simulink model "P702_NI_SoftECU"  (R2019a)
settings: Solver=ode1  StartTime=0.0  StopTime=Inf  FixedStep=0.001  RelTol=1e-3  EnableMultiTasking=on
PreLoadFcn:
  | run '.\VeriStand_BlockSet\NIVeriStandAddPaths.m'
undefined symbols (not defined in the file or in its folder): magnitude
libraries: simulink x83, simulink_extras x1
(part 40 of 76)

== system P702_NI_SoftECU/Output/SoftECULogic_NIXNET_CAN_FD1/WheelSpeed ==
  in : Inport
  WhlFl_W_Meas : S-Function  Priority=4  FunctionName=NIVeriStandIO  Parameters=width dtype portnum stime stype btype  SFunctionDeploymentMode=off  EnableBusSupport=off  mask(NI VeriStand Outport){portnum=4, width=-1, stime=-1, dtype=auto, stype=auto, btype=0}
      mask prompts: portnum "Port number:"; width "Port dimensions (-1 for dynamically sized):"; stime "Sample time (-1 for inherited):"; dtype "Data type:"; stype "Signal type:"; btype "Block type:"
      mask help: Use this outport on any level of nested subsystems to allow NI VeriStand software to map signals to it.
      mask init:
      | NIVeriStandIO_init;
      settings: CopyFcn=NIVeriStand_MDL_functions('', 'IO_copy');  DeleteFcn=NIVeriStand_MDL_functions('', 'IO_delete');  MoveFcn=set_param(gcb, 'Mask', 'on');
      mask Callback portnum: NIVeriStand_MDL_functions('', 'IO_setportnum');
      mask TypeOptions dtype: auto | double | single | int8 | uint8 | int16 | uint16 | int32 | uint32 | boolean
      mask Callback dtype: NIVeriStand_MDL_functions('', 'IO_booleansignal');
      mask TypeOptions stype: auto | real | complex
      mask Display:
      | patch([-x x], [-y y], [.90980 .81960 .32156]);
      | plot([xrad -x x xrad], [yrad -y y yrad]);
      | fprintf('NI Out%d', portnum);
  WhlFr_W_Meas : S-Function  Priority=3  FunctionName=NIVeriStandIO  Parameters=width dtype portnum stime stype btype  SFunctionDeploymentMode=off  EnableBusSupport=off  mask(NI VeriStand Outport){portnum=3, width=-1, stime=-1, dtype=auto, stype=auto, btype=0}
      mask prompts: portnum "Port number:"; width "Port dimensions (-1 for dynamically sized):"; stime "Sample time (-1 for inherited):"; dtype "Data type:"; stype "Signal type:"; btype "Block type:"
      mask help: Use this outport on any level of nested subsystems to allow NI VeriStand software to map signals to it.
      mask init:
      | NIVeriStandIO_init;
      settings: CopyFcn=NIVeriStand_MDL_functions('', 'IO_copy');  DeleteFcn=NIVeriStand_MDL_functions('', 'IO_delete');  MoveFcn=set_param(gcb, 'Mask', 'on');
      mask Callback portnum: NIVeriStand_MDL_functions('', 'IO_setportnum');
      mask TypeOptions dtype: auto | double | single | int8 | uint8 | int16 | uint16 | int32 | uint32 | boolean
      mask Callback dtype: NIVeriStand_MDL_functions('', 'IO_booleansignal');
      mask TypeOptions stype: auto | real | complex
      mask Display:
      | patch([-x x], [-y y], [.90980 .81960 .32156]);
      | plot([xrad -x x xrad], [yrad -y y yrad]);
      | fprintf('NI Out%d', portnum);
  WhlRl_W_Meas : S-Function  Priority=2  FunctionName=NIVeriStandIO  Parameters=width dtype portnum stime stype btype  SFunctionDeploymentMode=off  EnableBusSupport=off  mask(NI VeriStand Outport){portnum=2, width=-1, stime=-1, dtype=auto, stype=auto, btype=0}
      mask prompts: portnum "Port number:"; width "Port dimensions (-1 for dynamically sized):"; stime "Sample time (-1 for inherited):"; dtype "Data type:"; stype "Signal type:"; btype "Block type:"
      mask help: Use this outport on any level of nested subsystems to allow NI VeriStand software to map signals to it.
      mask init:
      | NIVeriStandIO_init;
      settings: CopyFcn=NIVeriStand_MDL_functions('', 'IO_copy');  DeleteFcn=NIVeriStand_MDL_functions('', 'IO_delete');  MoveFcn=set_param(gcb, 'Mask', 'on');
      mask Callback portnum: NIVeriStand_MDL_functions('', 'IO_setportnum');
      mask TypeOptions dtype: auto | double | single | int8 | uint8 | int16 | uint16 | int32 | uint32 | boolean
      mask Callback dtype: NIVeriStand_MDL_functions('', 'IO_booleansignal');
      mask TypeOptions stype: auto | real | complex
      mask Display:
      | patch([-x x], [-y y], [.90980 .81960 .32156]);
      | plot([xrad -x x xrad], [yrad -y y yrad]);
      | fprintf('NI Out%d', portnum);
  WhlRotatFl_No_Cnt : S-Function  Priority=5  FunctionName=NIVeriStandIO  Parameters=width dtype portnum stime stype btype  SFunctionDeploymentMode=off  EnableBusSupport=off  mask(NI VeriStand Outport){portnum=5, width=-1, stime=-1, dtype=auto, stype=auto, btype=0}
      mask prompts: portnum "Port number:"; width "Port dimensions (-1 for dynamically sized):"; stime "Sample time (-1 for inherited):"; dtype "Data type:"; stype "Signal type:"; btype "Block type:"
      mask help: Use this outport on any level of nested subsystems to allow NI VeriStand software to map signals to it.
      mask init:
      | NIVeriStandIO_init;
      settings: CopyFcn=NIVeriStand_MDL_functions('', 'IO_copy');  DeleteFcn=NIVeriStand_MDL_functions('', 'IO_delete');  MoveFcn=set_param(gcb, 'Mask', 'on');
      mask Callback portnum: NIVeriStand_MDL_functions('', 'IO_setportnum');
      mask TypeOptions dtype: auto | double | single | int8 | uint8 | int16 | uint16 | int32 | uint32 | boolean
      mask Callback dtype: NIVeriStand_MDL_functions('', 'IO_booleansignal');
      mask TypeOptions stype: auto | real | complex
      mask Display:
      | patch([-x x], [-y y], [.90980 .81960 .32156]);
      | plot([xrad -x x xrad], [yrad -y y yrad]);
      | fprintf('NI Out%d', portnum);
  WhlRotatFr_No_Cnt : S-Function  Priority=6  FunctionName=NIVeriStandIO  Parameters=width dtype portnum stime stype btype  SFunctionDeploymentMode=off  EnableBusSupport=off  mask(NI VeriStand Outport){portnum=6, width=-1, stime=-1, dtype=auto, stype=auto, btype=0}
      mask prompts: portnum "Port number:"; width "Port dimensions (-1 for dynamically sized):"; stime "Sample time (-1 for inherited):"; dtype "Data type:"; stype "Signal type:"; btype "Block type:"
      mask help: Use this outport on any level of nested subsystems to allow NI VeriStand software to map signals to it.
      mask init:
      | NIVeriStandIO_init;
      settings: CopyFcn=NIVeriStand_MDL_functions('', 'IO_copy');  DeleteFcn=NIVeriStand_MDL_functions('', 'IO_delete');  MoveFcn=set_param(gcb, 'Mask', 'on');
      mask Callback portnum: NIVeriStand_MDL_functions('', 'IO_setportnum');
      mask TypeOptions dtype: auto | double | single | int8 | uint8 | int16 | uint16 | int32 | uint32 | boolean
      mask Callback dtype: NIVeriStand_MDL_functions('', 'IO_booleansignal');
      mask TypeOptions stype: auto | real | complex
      mask Display:
      | patch([-x x], [-y y], [.90980 .81960 .32156]);
      | plot([xrad -x x xrad], [yrad -y y yrad]);
      | fprintf('NI Out%d', portnum);
  WhlRotatRl_No_Cnt : S-Function  Priority=7  FunctionName=NIVeriStandIO  Parameters=width dtype portnum stime stype btype  SFunctionDeploymentMode=off  EnableBusSupport=off  mask(NI VeriStand Outport){portnum=7, width=-1, stime=-1, dtype=auto, stype=auto, btype=0}
      mask prompts: portnum "Port number:"; width "Port dimensions (-1 for dynamically sized):"; stime "Sample time (-1 for inherited):"; dtype "Data type:"; stype "Signal type:"; btype "Block type:"
      mask help: Use this outport on any level of nested subsystems to allow NI VeriStand software to map signals to it.
      mask init:
      | NIVeriStandIO_init;
      settings: CopyFcn=NIVeriStand_MDL_functions('', 'IO_copy');  DeleteFcn=NIVeriStand_MDL_functions('', 'IO_delete');  MoveFcn=set_param(gcb, 'Mask', 'on');
      mask Callback portnum: NIVeriStand_MDL_functions('', 'IO_setportnum');
      mask TypeOptions dtype: auto | double | single | int8 | uint8 | int16 | uint16 | int32 | uint32 | boolean
      mask Callback dtype: NIVeriStand_MDL_functions('', 'IO_booleansignal');
      mask TypeOptions stype: auto | real | complex
      mask Display:
      | patch([-x x], [-y y], [.90980 .81960 .32156]);
      | plot([xrad -x x xrad], [yrad -y y yrad]);
      | fprintf('NI Out%d', portnum);
  WhlRotatRr_No_Cnt : S-Function  Priority=8  FunctionName=NIVeriStandIO  Parameters=width dtype portnum stime stype btype  SFunctionDeploymentMode=off  EnableBusSupport=off  mask(NI VeriStand Outport){portnum=8, width=-1, stime=-1, dtype=auto, stype=auto, btype=0}
      mask prompts: portnum "Port number:"; width "Port dimensions (-1 for dynamically sized):"; stime "Sample time (-1 for inherited):"; dtype "Data type:"; stype "Signal type:"; btype "Block type:"
      mask help: Use this outport on any level of nested subsystems to allow NI VeriStand software to map signals to it.
      mask init:
      | NIVeriStandIO_init;
      settings: CopyFcn=NIVeriStand_MDL_functions('', 'IO_copy');  DeleteFcn=NIVeriStand_MDL_functions('', 'IO_delete');  MoveFcn=set_param(gcb, 'Mask', 'on');
      mask Callback portnum: NIVeriStand_MDL_functions('', 'IO_setportnum');
      mask TypeOptions dtype: auto | double | single | int8 | uint8 | int16 | uint16 | int32 | uint32 | boolean
      mask Callback dtype: NIVeriStand_MDL_functions('', 'IO_booleansignal');
      mask TypeOptions stype: auto | real | complex
      mask Display:
      | patch([-x x], [-y y], [.90980 .81960 .32156]);
      | plot([xrad -x x xrad], [yrad -y y yrad]);
      | fprintf('NI Out%d', portnum);
  WhlRr_W_Meas : S-Function  Priority=1  FunctionName=NIVeriStandIO  Parameters=width dtype portnum stime stype btype  SFunctionDeploymentMode=off  EnableBusSupport=off  mask(NI VeriStand Outport){portnum=1, width=-1, stime=-1, dtype=auto, stype=auto, btype=0}
      mask prompts: portnum "Port number:"; width "Port dimensions (-1 for dynamically sized):"; stime "Sample time (-1 for inherited):"; dtype "Data type:"; stype "Signal type:"; btype "Block type:"
      mask help: Use this outport on any level of nested subsystems to allow NI VeriStand software to map signals to it.
      mask init:
      | NIVeriStandIO_init;
      settings: CopyFcn=NIVeriStand_MDL_functions('', 'IO_copy');  DeleteFcn=NIVeriStand_MDL_functions('', 'IO_delete');  MoveFcn=set_param(gcb, 'Mask', 'on');
      mask Callback portnum: NIVeriStand_MDL_functions('', 'IO_setportnum');
      mask TypeOptions dtype: auto | double | single | int8 | uint8 | int16 | uint16 | int32 | uint32 | boolean
      mask Callback dtype: NIVeriStand_MDL_functions('', 'IO_booleansignal');
      mask TypeOptions stype: auto | real | complex
      mask Display:
      | patch([-x x], [-y y], [.90980 .81960 .32156]);
      | plot([xrad -x x xrad], [yrad -y y yrad]);
      | fprintf('NI Out%d', portnum);
  busselector : BusSelector  OutputSignals=Soft_ABS.WheelSpeed.WhlRr_W_Meas,Soft_ABS.WheelSpeed.WhlRl_W_Meas,Soft_ABS.WheelSpeed.WhlFr_W_Meas,Soft_ABS.WheelSpeed.WhlFl_W_Meas,Soft_ABS.WheelSpeed.WhlRotatFl_No_Cnt,Soft_ABS.WheelSpeed.WhlRotatFr_No_Cnt,Soft_ABS.WheelSpeed.WhlRotatRl_No_Cnt,Soft_ABS.WheelSpeed.WhlRotatRr_No_Cnt
  dt_WhlFl_W_Meas{,1..4} (5 alike) : DataTypeConversion  RndMeth=Zero
  dt_WhlFr_W_Meas : DataTypeConversion  RndMeth=Zero
  dt_WhlRl_W_Meas : DataTypeConversion  RndMeth=Zero
  dt_WhlRr_W_Meas : DataTypeConversion  RndMeth=Zero
  wires:
  in/1 -> busselector/1
  busselector/1 -> dt_WhlRr_W_Meas/1  "<WhlRr_W_Meas>"
  dt_WhlRr_W_Meas/1 -> WhlRr_W_Meas/1  "WhlRr_W_Meas"
  busselector/2 -> dt_WhlRl_W_Meas/1  "<WhlRl_W_Meas>"
  dt_WhlRl_W_Meas/1 -> WhlRl_W_Meas/1  "WhlRl_W_Meas"
  busselector/3 -> dt_WhlFr_W_Meas/1  "<WhlFr_W_Meas>"
  dt_WhlFr_W_Meas/1 -> WhlFr_W_Meas/1  "WhlFr_W_Meas"
  busselector/4 -> dt_WhlFl_W_Meas/1  "<WhlFl_W_Meas>"
  dt_WhlFl_W_Meas/1 -> WhlFl_W_Meas/1  "WhlFl_W_Meas"
  dt_WhlFl_W_Meas1/1 -> WhlRotatFr_No_Cnt/1  "<WhlRotatFr_No_Cnt>"
  dt_WhlFl_W_Meas2/1 -> WhlRotatFl_No_Cnt/1  "<WhlRotatFl_No_Cnt>"
  dt_WhlFl_W_Meas3/1 -> WhlRotatRr_No_Cnt/1  "<WhlRotatRr_No_Cnt>"
  dt_WhlFl_W_Meas4/1 -> WhlRotatRl_No_Cnt/1  "<WhlRotatRl_No_Cnt>"
  busselector/7 -> dt_WhlFl_W_Meas3/1  "<WhlRotatRl_No_Cnt>"
  busselector/6 -> dt_WhlFl_W_Meas2/1  "<WhlRotatFr_No_Cnt>"
  busselector/5 -> dt_WhlFl_W_Meas1/1  "<WhlRotatFl_No_Cnt>"
  busselector/8 -> dt_WhlFl_W_Meas4/1  "<WhlRotatRr_No_Cnt>"

== system P702_NI_SoftECU/Output/SoftECULogic_NIXNET_CAN_FD1/Yaw_Data ==
  in : Inport
  VehRolWActl_D_Qf : S-Function  Priority=2  FunctionName=NIVeriStandIO  Parameters=width dtype portnum stime stype btype  SFunctionDeploymentMode=off  EnableBusSupport=off  mask(NI VeriStand Outport){portnum=2, width=-1, stime=-1, dtype=auto, stype=auto, btype=0}
      mask prompts: portnum "Port number:"; width "Port dimensions (-1 for dynamically sized):"; stime "Sample time (-1 for inherited):"; dtype "Data type:"; stype "Signal type:"; btype "Block type:"
      mask help: Use this outport on any level of nested subsystems to allow NI VeriStand software to map signals to it.
      mask init:
      | NIVeriStandIO_init;
      settings: CopyFcn=NIVeriStand_MDL_functions('', 'IO_copy');  DeleteFcn=NIVeriStand_MDL_functions('', 'IO_delete');  MoveFcn=set_param(gcb, 'Mask', 'on');
      mask Callback portnum: NIVeriStand_MDL_functions('', 'IO_setportnum');
      mask TypeOptions dtype: auto | double | single | int8 | uint8 | int16 | uint16 | int32 | uint32 | boolean
      mask Callback dtype: NIVeriStand_MDL_functions('', 'IO_booleansignal');
      mask TypeOptions stype: auto | real | complex
      mask Display:
      | patch([-x x], [-y y], [.90980 .81960 .32156]);
      | plot([xrad -x x xrad], [yrad -y y yrad]);
      | fprintf('NI Out%d', portnum);
  VehRol_W_Actl : S-Function  Priority=3  FunctionName=NIVeriStandIO  Parameters=width dtype portnum stime stype btype  SFunctionDeploymentMode=off  EnableBusSupport=off  mask(NI VeriStand Outport){portnum=3, width=-1, stime=-1, dtype=auto, stype=auto, btype=0}
      mask prompts: portnum "Port number:"; width "Port dimensions (-1 for dynamically sized):"; stime "Sample time (-1 for inherited):"; dtype "Data type:"; stype "Signal type:"; btype "Block type:"
      mask help: Use this outport on any level of nested subsystems to allow NI VeriStand software to map signals to it.
      mask init:
      | NIVeriStandIO_init;
      settings: CopyFcn=NIVeriStand_MDL_functions('', 'IO_copy');  DeleteFcn=NIVeriStand_MDL_functions('', 'IO_delete');  MoveFcn=set_param(gcb, 'Mask', 'on');
      mask Callback portnum: NIVeriStand_MDL_functions('', 'IO_setportnum');
      mask TypeOptions dtype: auto | double | single | int8 | uint8 | int16 | uint16 | int32 | uint32 | boolean
      mask Callback dtype: NIVeriStand_MDL_functions('', 'IO_booleansignal');
      mask TypeOptions stype: auto | real | complex
      mask Display:
      | patch([-x x], [-y y], [.90980 .81960 .32156]);
      | plot([xrad -x x xrad], [yrad -y y yrad]);
      | fprintf('NI Out%d', portnum);
  VehRollYawW_No_Cs : S-Function  Priority=4  FunctionName=NIVeriStandIO  Parameters=width dtype portnum stime stype btype  SFunctionDeploymentMode=off  EnableBusSupport=off  mask(NI VeriStand Outport){portnum=4, width=-1, stime=-1, dtype=auto, stype=auto, btype=0}
      mask prompts: portnum "Port number:"; width "Port dimensions (-1 for dynamically sized):"; stime "Sample time (-1 for inherited):"; dtype "Data type:"; stype "Signal type:"; btype "Block type:"
      mask help: Use this outport on any level of nested subsystems to allow NI VeriStand software to map signals to it.
      mask init:
      | NIVeriStandIO_init;
      settings: CopyFcn=NIVeriStand_MDL_functions('', 'IO_copy');  DeleteFcn=NIVeriStand_MDL_functions('', 'IO_delete');  MoveFcn=set_param(gcb, 'Mask', 'on');
      mask Callback portnum: NIVeriStand_MDL_functions('', 'IO_setportnum');
      mask TypeOptions dtype: auto | double | single | int8 | uint8 | int16 | uint16 | int32 | uint32 | boolean
      mask Callback dtype: NIVeriStand_MDL_functions('', 'IO_booleansignal');
      mask TypeOptions stype: auto | real | complex
      mask Display:
      | patch([-x x], [-y y], [.90980 .81960 .32156]);
      | plot([xrad -x x xrad], [yrad -y y yrad]);
      | fprintf('NI Out%d', portnum);
  VehRollYaw_No_Cnt : S-Function  Priority=5  FunctionName=NIVeriStandIO  Parameters=width dtype portnum stime stype btype  SFunctionDeploymentMode=off  EnableBusSupport=off  mask(NI VeriStand Outport){portnum=5, width=-1, stime=-1, dtype=auto, stype=auto, btype=0}
      mask prompts: portnum "Port number:"; width "Port dimensions (-1 for dynamically sized):"; stime "Sample time (-1 for inherited):"; dtype "Data type:"; stype "Signal type:"; btype "Block type:"
      mask help: Use this outport on any level of nested subsystems to allow NI VeriStand software to map signals to it.
      mask init:
      | NIVeriStandIO_init;
      settings: CopyFcn=NIVeriStand_MDL_functions('', 'IO_copy');  DeleteFcn=NIVeriStand_MDL_functions('', 'IO_delete');  MoveFcn=set_param(gcb, 'Mask', 'on');
      mask Callback portnum: NIVeriStand_MDL_functions('', 'IO_setportnum');
      mask TypeOptions dtype: auto | double | single | int8 | uint8 | int16 | uint16 | int32 | uint32 | boolean
      mask Callback dtype: NIVeriStand_MDL_functions('', 'IO_booleansignal');
      mask TypeOptions stype: auto | real | complex
      mask Display:
      | patch([-x x], [-y y], [.90980 .81960 .32156]);
      | plot([xrad -x x xrad], [yrad -y y yrad]);
      | fprintf('NI Out%d', portnum);
  VehYawWActl_D_Qf : S-Function  Priority=6  FunctionName=NIVeriStandIO  Parameters=width dtype portnum stime stype btype  SFunctionDeploymentMode=off  EnableBusSupport=off  mask(NI VeriStand Outport){portnum=6, width=-1, stime=-1, dtype=auto, stype=auto, btype=0}
      mask prompts: portnum "Port number:"; width "Port dimensions (-1 for dynamically sized):"; stime "Sample time (-1 for inherited):"; dtype "Data type:"; stype "Signal type:"; btype "Block type:"
      mask help: Use this outport on any level of nested subsystems to allow NI VeriStand software to map signals to it.
      mask init:
      | NIVeriStandIO_init;
      settings: CopyFcn=NIVeriStand_MDL_functions('', 'IO_copy');  DeleteFcn=NIVeriStand_MDL_functions('', 'IO_delete');  MoveFcn=set_param(gcb, 'Mask', 'on');
      mask Callback portnum: NIVeriStand_MDL_functions('', 'IO_setportnum');
      mask TypeOptions dtype: auto | double | single | int8 | uint8 | int16 | uint16 | int32 | uint32 | boolean
      mask Callback dtype: NIVeriStand_MDL_functions('', 'IO_booleansignal');
      mask TypeOptions stype: auto | real | complex
      mask Display:
      | patch([-x x], [-y y], [.90980 .81960 .32156]);
      | plot([xrad -x x xrad], [yrad -y y yrad]);
      | fprintf('NI Out%d', portnum);
  VehYaw_W_Actl : S-Function  Priority=1  FunctionName=NIVeriStandIO  Parameters=width dtype portnum stime stype btype  SFunctionDeploymentMode=off  EnableBusSupport=off  mask(NI VeriStand Outport){portnum=1, width=-1, stime=-1, dtype=auto, stype=auto, btype=0}
      mask prompts: portnum "Port number:"; width "Port dimensions (-1 for dynamically sized):"; stime "Sample time (-1 for inherited):"; dtype "Data type:"; stype "Signal type:"; btype "Block type:"
      mask help: Use this outport on any level of nested subsystems to allow NI VeriStand software to map signals to it.
      mask init:
      | NIVeriStandIO_init;
      settings: CopyFcn=NIVeriStand_MDL_functions('', 'IO_copy');  DeleteFcn=NIVeriStand_MDL_functions('', 'IO_delete');  MoveFcn=set_param(gcb, 'Mask', 'on');
      mask Callback portnum: NIVeriStand_MDL_functions('', 'IO_setportnum');
      mask TypeOptions dtype: auto | double | single | int8 | uint8 | int16 | uint16 | int32 | uint32 | boolean
      mask Callback dtype: NIVeriStand_MDL_functions('', 'IO_booleansignal');
      mask TypeOptions stype: auto | real | complex
      mask Display:
      | patch([-x x], [-y y], [.90980 .81960 .32156]);
      | plot([xrad -x x xrad], [yrad -y y yrad]);
      | fprintf('NI Out%d', portnum);
  busselector : BusSelector  OutputSignals=Soft_RCM.Yaw_Data.VehYawWActl_D_Qf,Soft_RCM.Yaw_Data.VehRolWActl_D_Qf,Soft_RCM.Yaw_Data.VehRollYaw_No_Cnt,Soft_RCM.Yaw_Data.VehRollYawW_No_Cs,Soft_RCM.Yaw_Data.VehYaw_W_Actl,Soft_RCM.Yaw_Data.VehRol_W_Actl
  dt_VehRolWActl_D_Qf : DataTypeConversion  RndMeth=Zero
  dt_VehRol_W_Actl : DataTypeConversion  RndMeth=Zero
  dt_VehRollYawW_No_Cs : DataTypeConversion  RndMeth=Zero
  dt_VehRollYaw_No_Cnt : DataTypeConversion  RndMeth=Zero
  dt_VehYawWActl_D_Qf : DataTypeConversion  RndMeth=Zero
  dt_VehYaw_W_Actl : DataTypeConversion  RndMeth=Zero
  wires:
  in/1 -> busselector/1
  busselector/1 -> dt_VehYawWActl_D_Qf/1  "<VehYawWActl_D_Qf>"
  dt_VehYawWActl_D_Qf/1 -> VehYawWActl_D_Qf/1  "VehYawWActl_D_Qf"
  busselector/2 -> dt_VehRolWActl_D_Qf/1  "<VehRolWActl_D_Qf>"
  dt_VehRolWActl_D_Qf/1 -> VehRolWActl_D_Qf/1  "VehRolWActl_D_Qf"
  busselector/3 -> dt_VehRollYaw_No_Cnt/1  "<VehRollYaw_No_Cnt>"
  dt_VehRollYaw_No_Cnt/1 -> VehRollYaw_No_Cnt/1  "VehRollYaw_No_Cnt"
  busselector/4 -> dt_VehRollYawW_No_Cs/1  "<VehRollYawW_No_Cs>"
  dt_VehRollYawW_No_Cs/1 -> VehRollYawW_No_Cs/1  "VehRollYawW_No_Cs"
  busselector/5 -> dt_VehYaw_W_Actl/1  "<VehYaw_W_Actl>"
  dt_VehYaw_W_Actl/1 -> VehYaw_W_Actl/1  "VehYaw_W_Actl"
  busselector/6 -> dt_VehRol_W_Actl/1  "<VehRol_W_Actl>"
  dt_VehRol_W_Actl/1 -> VehRol_W_Actl/1  "VehRol_W_Actl"

== system P702_NI_SoftECU/Output/Subsystem/a//b ==
  Constant : Constant
  x/y : Constant
  Out1 : Outport
  wires:
  Constant/1 -> Out1/1

== system P702_NI_SoftECU/Output/Subsystem/c ==
  In1 : Inport
  Out1 : Outport
  wires:
  In1/1 -> Out1/1

== system P702_NI_SoftECU/Output/Subsystem/d ==
  In1 : Inport
  Out1 : Outport
  wires:
  In1/1 -> Out1/1

== system P702_NI_SoftECU/Output/Subsystem1/CAN_Signal ==
  in_port : Inport
  ABS_ESC : Subsystem
  ADAS : Subsystem
  BCM : Subsystem
  DSMC : Subsystem
  ECM_DIESEL PCM PCM_HEV : Subsystem
  GWM : Subsystem
  PSCM : Subsystem
  RealPCM : Subsystem
  bus_selector : BusSelector  OutputSignals=ADAS,RealPCM,ABS_ESC,PSCM,ECM_DIESEL PCM PCM_HEV,BCM,GWM,DSMC
  wires:
  in_port/1 -> bus_selector/1  "Subsystem1"
  bus_selector/1 -> ADAS/1(in_port)  "<ADAS>"
  bus_selector/2 -> RealPCM/1(in_port)  "<RealPCM>"
  bus_selector/3 -> ABS_ESC/1(in_port)  "<ABS_ESC>"
  bus_selector/4 -> PSCM/1(in_port)  "<PSCM>"
  bus_selector/5 -> ECM_DIESEL PCM PCM_HEV/1(in_port)  "<ECM_DIESEL PCM PCM_HEV>"
  bus_selector/6 -> BCM/1(in_port)  "<BCM>"
  bus_selector/7 -> GWM/1(in_port)  "<GWM>"
  bus_selector/8 -> DSMC/1(in_port)  "<DSMC>"

== system P702_NI_SoftECU/Output/Subsystem1/To_NI_HIL ==
  in_port : Inport
  DSMC : Subsystem
  MRR : Subsystem
  SRR_L : Subsystem
  SRR_R : Subsystem
  Soft_ABS : Subsystem
  Soft_APIM : Terminator
  Soft_BCM : Subsystem
  Soft_CCM : Terminator
  Soft_ECM : Subsystem
  Soft_IPC : Terminator
  Soft_IPMA : Terminator
  Soft_MRR : Subsystem
  Soft_PCM : Subsystem
  Soft_PSCM : Subsystem
  Soft_RCM : Subsystem
  Soft_SCCM : Subsystem
  Soft_TCM : Subsystem
  bus_selector : BusSelector  OutputSignals=Soft_ABS,Soft_PCM,Soft_ECM,Soft_TCM,Soft_PSCM,Soft_RCM,Soft_SCCM,Soft_MRR,Soft_BCM,Soft_IPC,Soft_APIM,Soft_IPMA,Soft_CCM,MRR,SRR_R,SRR_L,DSMC
  wires:
  in_port/1 -> bus_selector/1  "Subsystem1"
  bus_selector/10 -> Soft_IPC/1  "<Soft_IPC>"
  bus_selector/11 -> Soft_APIM/1  "<Soft_APIM>"
  bus_selector/12 -> Soft_IPMA/1  "<Soft_IPMA>"
  bus_selector/13 -> Soft_CCM/1  "<Soft_CCM>"
  bus_selector/1 -> Soft_ABS/1(in_port)  "<Soft_ABS>"
  bus_selector/2 -> Soft_PCM/1(in_port)  "<Soft_PCM>"
  bus_selector/3 -> Soft_ECM/1(in_port)  "<Soft_ECM>"
  bus_selector/4 -> Soft_TCM/1(in_port)  "<Soft_TCM>"
  bus_selector/5 -> Soft_PSCM/1(in_port)  "<Soft_PSCM>"
  bus_selector/6 -> Soft_RCM/1(in_port)  "<Soft_RCM>"
  bus_selector/7 -> Soft_SCCM/1(in_port)  "<Soft_SCCM>"
  bus_selector/8 -> Soft_MRR/1(in_port)  "<Soft_MRR>"
  bus_selector/9 -> Soft_BCM/1(in_port)  "<Soft_BCM>"
  bus_selector/14 -> MRR/1(in_port)  "<MRR>"
  bus_selector/15 -> SRR_R/1(in_port)  "<SRR_R>"
  bus_selector/16 -> SRR_L/1(in_port)  "<SRR_L>"
  bus_selector/17 -> DSMC/1(in_port)  "<DSMC>"

== system P702_NI_SoftECU/Output/Subsystem2/CAN_Signal ==
  ABS_ESC : Subsystem
  ADAS : Subsystem
  BCM : Subsystem
  DSMC : Subsystem
  ECM_DIESEL PCM PCM_HEV : Subsystem
  GWM : Subsystem
  PSCM : Subsystem
  RealPCM : Subsystem
  bus_creator : BusCreator  Inputs=8
  out_port : Outport
  wires:
  bus_creator/1 -> out_port/1  "Subsystem2"
  ADAS/1(out_port) -> bus_creator/1  "ADAS"
  RealPCM/1(out_port) -> bus_creator/2  "RealPCM"
  ABS_ESC/1(out_port) -> bus_creator/3  "ABS_ESC"
  PSCM/1(out_port) -> bus_creator/4  "PSCM"
  ECM_DIESEL PCM PCM_HEV/1(out_port) -> bus_creator/5  "ECM_DIESEL PCM PCM_HEV"
  BCM/1(out_port) -> bus_creator/6  "BCM"
  GWM/1(out_port) -> bus_creator/7  "GWM"
  DSMC/1(out_port) -> bus_creator/8  "DSMC"

== system P702_NI_SoftECU/Output/Subsystem2/To_NI_HIL ==
  DSMC : Subsystem
  MRR : Subsystem
  SRR_L : Subsystem
  SRR_R : Subsystem
  Soft_ABS : Subsystem
  Soft_APIM : Constant  Value=0
  Soft_BCM : Subsystem
  Soft_CCM : Constant  Value=0
  Soft_ECM : Subsystem
  Soft_IPC : Constant  Value=0
  Soft_IPMA : Constant  Value=0
  Soft_MRR : Subsystem
  Soft_PCM : Subsystem
  Soft_PSCM : Subsystem
  Soft_RCM : Subsystem
  Soft_SCCM : Subsystem
  Soft_TCM : Subsystem
  bus_creator : BusCreator  Inputs=17
  out_port : Outport
  wires:
  bus_creator/1 -> out_port/1  "Subsystem2"
  Soft_IPC/1 -> bus_creator/10  "Soft_IPC"
  Soft_APIM/1 -> bus_creator/11  "Soft_APIM"
  Soft_IPMA/1 -> bus_creator/12  "Soft_IPMA"
  Soft_CCM/1 -> bus_creator/13  "Soft_CCM"
  Soft_ABS/1(out_port) -> bus_creator/1  "Soft_ABS"
  Soft_PCM/1(out_port) -> bus_creator/2  "Soft_PCM"
  Soft_ECM/1(out_port) -> bus_creator/3  "Soft_ECM"
  Soft_TCM/1(out_port) -> bus_creator/4  "Soft_TCM"
  Soft_PSCM/1(out_port) -> bus_creator/5  "Soft_PSCM"
  Soft_RCM/1(out_port) -> bus_creator/6  "Soft_RCM"
  Soft_SCCM/1(out_port) -> bus_creator/7  "Soft_SCCM"
  Soft_MRR/1(out_port) -> bus_creator/8  "Soft_MRR"
  Soft_BCM/1(out_port) -> bus_creator/9  "Soft_BCM"
  MRR/1(out_port) -> bus_creator/14  "MRR"
  SRR_R/1(out_port) -> bus_creator/15  "SRR_R"
  SRR_L/1(out_port) -> bus_creator/16  "SRR_L"
  DSMC/1(out_port) -> bus_creator/17  "DSMC"

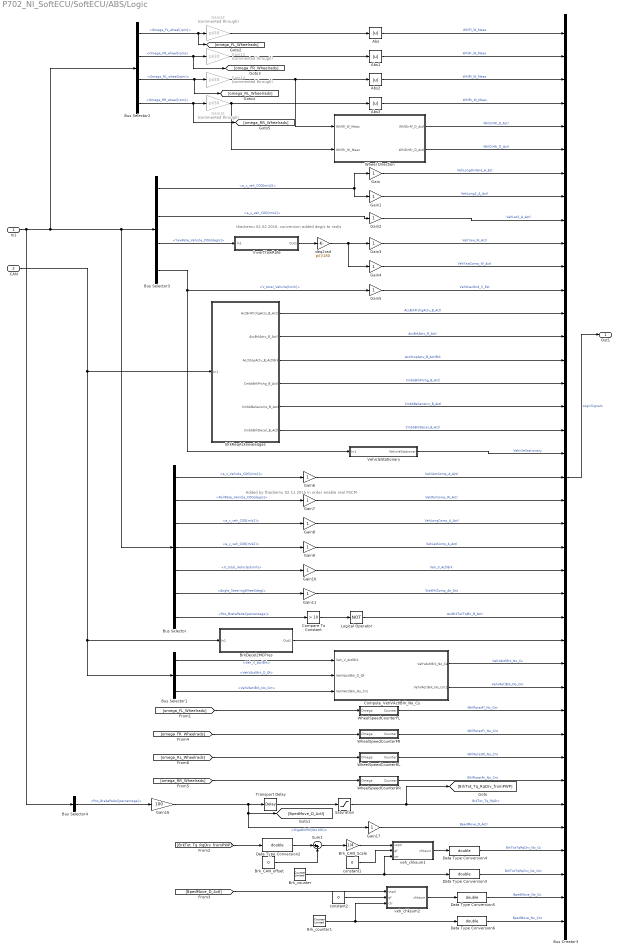
== system P702_NI_SoftECU/SoftECU/ABS/Logic ==
  note: thackemu 02.02.2016: conversion added deg/s to rad/s
  note: Added by thackemu 02.11.2015 in order enable real PSCM
  In1 : Inport
  CAN : Inport  Port=2
  Abs{,1..3} (4 alike) : Abs
  BrkDecel2MCPres : Subsystem
  BrkReqAcknowledges : Subsystem
  Brk_CAN_Scale : Gain  Gain=1/4
  Brk_CAN_offset : Constant  Value=0
  Brk_counter : simulink/Sources/Counter Limited  uplimit=15  tsamp=-1
  Brk_counter1 : simulink/Sources/Counter Limited  uplimit=15  tsamp=-1
  Bus Creator3 : BusCreator  Inputs=39
  Bus Selector : BusSelector  OutputSignals=a_z_Vehicle_COG[m/s2],RollRate_Vehicle_COG[deg/s],a_x_veh_COG[m/s2],a_y_veh_COG[m/s2],V_total_Vehicle[km/h],Angle_SteeringWheel[deg],Pos_BrakePedal[percentage]
  Bus Selector1 : BusSelector  OutputSignals=ABS_ESC.BrakeSysFeatures_0x415.Veh_V_ActlBrk,ABS_ESC.BrakeSysFeatures_0x415.VehVActlBrk_D_Qf,ABS_ESC.BrakeSysFeatures_0x415.VehVActlBrk_No_Cnt
  Bus Selector2 : BusSelector  OutputSignals=Omega_FL_wheel[rpm],Omega_FR_wheel[rpm],Omega_RL_wheel[rpm],Omega_RR_wheel[rpm]
  Bus Selector3 : BusSelector  OutputSignals=a_x_veh_COG[m/s2],a_y_veh_COG[m/s2],YawRate_Vehicle_COG[deg/s],V_total_Vehicle[km/h]
  Bus Selector4 : BusSelector  OutputSignals=Pos_BrakePedal[percentage]
  Compare To Constant : simulink/Logic and Bit Operations/Compare To Constant  relop=>  const=10  OutDataTypeStr=boolean
  Compute_VehVActlBrk_No_Cs : Subsystem
  Data Type Conversion{2..6} (5 alike) : DataTypeConversion  OutDataTypeStr=double
  Gain{,1..11,17} (13 alike) : Gain
  Gain{12..15} (4 alike) : Gain  Commented=through  Gain=pi/30
  Gain16 : Gain  Gain=100
  InvertYawRate : Subsystem
  Logical Operator : Logic  Operator=NOT  AllPortsSameDT=off  OutDataTypeStr=boolean
  Saturation : Saturate  UpperLimit=2000  LowerLimit=0
  Sum1 : Sum  Inputs=|++
  Transport Delay : TransportDelay  DelayTime=0.2  BufferSize=25600  FixedBuffer=on  TransDelayFeedthrough=on
  VehicleStationary : Subsystem
  Wheel Direction : Subsystem
  WheelSpeedCounterFL : Subsystem
  WheelSpeedCounterFR : Subsystem
  WheelSpeedCounterRL : Subsystem
  WheelSpeedCounterRR : Subsystem
  constant1 : Constant  Value=0
  constant2 : Constant  Value=0
  deg2rad : Gain  Gain=pi()/180
  veh_chksum1 : Subsystem
  veh_chksum2 : Subsystem
  Out1 : Outport
  wires:
  Bus Creator3/1 -> Out1/1  "LogicSignals"
  Bus Selector2/1 -> [omega_FL_Wheelrads], Gain12/1  "<Omega_FL_wheel[rpm]>"
  Bus Selector2/2 -> [omega_FR_Wheelrads], Gain13/1  "<Omega_FR_wheel[rpm]>"
  Bus Selector2/3 -> [omega_RL_Wheelrads], Gain14/1  "<Omega_RL_wheel[rpm]>"
  Abs/1 -> Bus Creator3/1  "WhlFl_W_Meas"
  Abs1/1 -> Bus Creator3/2  "WhlFr_W_Meas"
  Abs2/1 -> Bus Creator3/3  "WhlRl_W_Meas"
  Abs3/1 -> Bus Creator3/4  "WhlRr_W_Meas"
  Bus Selector2/4 -> [omega_RR_Wheelrads], Gain15/1  "<Omega_RR_wheel[rpm]>"
  Bus Selector3/2 -> Gain2/1  "<a_y_veh_COG[m/s2]>"
  Bus Selector3/4 -> Gain5/1, VehicleStationary/1(In1)  "<V_total_Vehicle[km/h]>"
  Gain1/1 -> Bus Creator3/8  "VehLong2_A_Actl"
  Gain2/1 -> Bus Creator3/9  "VehLat2_A_Actl"
  Gain3/1 -> Bus Creator3/10  "VehYaw_W_Actl"
  Gain/1 -> Bus Creator3/7  "VehLongOvrGnd_A_Est"
  Gain5/1 -> Bus Creator3/12  "VehOverGnd_V_Est"
  Gain4/1 -> Bus Creator3/11  "VehYawComp_W_Actl"
  Gain6/1 -> Bus Creator3/20  "VehVertComp_A_Actl"
  Gain8/1 -> Bus Creator3/22  "VehLongComp_A_Actl"
  Gain9/1 -> Bus Creator3/23  "VehLatComp_A_Actl"
  Bus Selector/1 -> Gain6/1  "<a_z_Vehicle_COG[m/s2]>"
  Gain7/1 -> Bus Creator3/21  "VehRolComp_W_Actl"
  Bus Selector/2 -> Gain7/1  "<RollRate_Vehicle_COG[deg/s]>"
  Gain10/1 -> Bus Creator3/24  "Veh_V_ActlBrk"
  BrkReqAcknowledges/2(AccBrkActv_B_Actl) -> Bus Creator3/14  "AccBrkActv_B_Actl"
  BrkReqAcknowledges/1(AccBrkPrchgActv_B_Actl) -> Bus Creator3/13  "AccBrkPrchgActv_B_Actl"
  BrkReqAcknowledges/3(AccStopActv_B_ActlBrk) -> Bus Creator3/15  "AccStopActv_B_ActlBrk"
  BrkReqAcknowledges/4(CmbbBrkPrchg_B_Actl) -> Bus Creator3/16  "CmbbBrkPrchg_B_Actl"
  BrkReqAcknowledges/5(CmbbBaSensInc_B_Actl) -> Bus Creator3/17  "CmbbBaSensInc_B_Actl"
  BrkReqAcknowledges/6(CmbbBrkDecel_B_Actl) -> Bus Creator3/18  "CmbbBrkDecel_B_Actl"
  VehicleStationary/1(VehicleStationary) -> Bus Creator3/19  "VehicleStationary"
  deg2rad/1 -> Gain4/1, Gain3/1
  Bus Selector3/3 -> InvertYawRate/1(In1)  "<YawRate_Vehicle_COG[deg/s]>"
  InvertYawRate/1(Out1) -> deg2rad/1
  Wheel Direction/1(WhlDirRl_D_Actl) -> Bus Creator3/5  "WhlDirRl_D_Actl"
  Wheel Direction/2(WhlDirRr_D_Actl) -> Bus Creator3/6  "WhlDirRr_D_Actl"
  Bus Selector3/1 -> Gain1/1, Gain/1  "<a_x_veh_COG[m/s2]>"
  Gain11/1 -> Bus Creator3/25  "SteWhlComp_An_Est"
  Compare To Constant/1 -> Logical Operator/1
  Logical Operator/1 -> Bus Creator3/26  "AccBrkTotTqMn_B_Actl"
  In1/1 -> Bus Selector4/1, Bus Selector2/1, Bus Selector/1, Bus Selector3/1
  Gain12/1 -> Abs/1
  Gain13/1 -> Abs1/1
  Gain14/1 -> Wheel Direction/1(WhlRl_W_Meas), Abs2/1
  Gain15/1 -> Wheel Direction/2(WhlRr_W_Meas), Abs3/1
  CAN/1 -> BrkReqAcknowledges/1(In1), Bus Selector1/1, BrkDecel2MCPres/1(In1)
  Bus Selector/3 -> Gain8/1  "<a_x_veh_COG[m/s2]>"
  Bus Selector/4 -> Gain9/1  "<a_y_veh_COG[m/s2]>"
  Bus Selector/5 -> Gain10/1  "<V_total_Vehicle[km/h]>"
  Bus Selector/6 -> Gain11/1  "<Angle_SteeringWheel[deg]>"
  Bus Selector/7 -> Compare To Constant/1  "<Pos_BrakePedal[percentage]>"
  BrkDecel2MCPres/1(Out1) -> Bus Creator3/27
  Bus Selector1/1 -> Compute_VehVActlBrk_No_Cs/1(Veh_V_ActlBrk)  "<Veh_V_ActlBrk>"
  Bus Selector1/2 -> Compute_VehVActlBrk_No_Cs/2(VehVActlBrk_D_Qf)  "<VehVActlBrk_D_Qf>"
  Bus Selector1/3 -> Compute_VehVActlBrk_No_Cs/3(VehVActlBrk_No_Cnt)  "<VehVActlBrk_No_Cnt>"
  Compute_VehVActlBrk_No_Cs/1(VehVActlBrk_No_Cs) -> Bus Creator3/28  "VehVActlBrk_No_Cs"
  Compute_VehVActlBrk_No_Cs/2(VehVActlBrk_No_Cnt1) -> Bus Creator3/29  "VehVActlBrk_No_Cnt"
  WheelSpeedCounterFL/1(Counter) -> Bus Creator3/30  "WhlRotatFl_No_Cnt"
  [omega_FL_Wheelrads] -> WheelSpeedCounterFL/1(Omega)
  [omega_RR_Wheelrads] -> WheelSpeedCounterRR/1(Omega)
  WheelSpeedCounterFR/1(Counter) -> Bus Creator3/31  "WhlRotatFr_No_Cnt"
  [omega_RL_Wheelrads] -> WheelSpeedCounterRL/1(Omega)
  WheelSpeedCounterRL/1(Counter) -> Bus Creator3/32  "WhlRotatRl_No_Cnt"
  WheelSpeedCounterRR/1(Counter) -> Bus Creator3/33  "WhlRotatRr_No_Cnt"
  [omega_FR_Wheelrads] -> WheelSpeedCounterFR/1(Omega)
  Bus Selector4/1 -> Gain16/1  "<Pos_BrakePedal[percentage]>"
  Transport Delay/1 -> Saturation/1
  Gain16/1 -> Gain17/1, [BpedMove_D_Actl], Transport Delay/1  "<GigaBrkPdl[0to10K]>"
  Gain17/1 -> Bus Creator3/35  "BpedMove_D_Actl"
  Saturation/1 -> Bus Creator3/34, [BrkTot_Tq_RqDrv_fromPWP]  "BrkTot_Tq_RqDrv"
  veh_chksum1/1(chksum) -> Data Type Conversion4/1
  veh_chksum2/1(chksum) -> Data Type Conversion5/1
  Data Type Conversion5/1 -> Bus Creator3/38  "BpedMove_No_Cs"
  constant1/1 -> veh_chksum1/2(qf)
  [BrkTot_Tq_RqDrv_fromPWP] -> Data Type Conversion2/1
  Data Type Conversion2/1 -> Sum1/1
  Sum1/1 -> Brk_CAN_Scale/1
  Brk_counter1/1 -> veh_chksum2/3(ctr), Data Type Conversion6/1
  Data Type Conversion3/1 -> Bus Creator3/37  "BrkTotTqRqDrv_No_Cnt"
  Data Type Conversion6/1 -> Bus Creator3/39  "BpedMove_No_Cnt"
  constant2/1 -> veh_chksum2/2(qf)
  Brk_CAN_offset/1 -> Sum1/2
  Brk_counter/1 -> veh_chksum1/3(ctr), Data Type Conversion3/1
  Data Type Conversion4/1 -> Bus Creator3/36  "BrkTotTqRqDrv_No_Cs"
  [BpedMove_D_Actl] -> veh_chksum2/1(vspd)
  Brk_CAN_Scale/1 -> veh_chksum1/1(vspd)

== system P702_NI_SoftECU/SoftECU/ABS/Mapping ==
  In1 : Inport
  ABS_BrkBst_Data : Subsystem
  Accel_Data : Subsystem
  BrakeSnData_3 : Subsystem
  BrakeSnData_4 : Subsystem
  BrakeSnData_5 : Subsystem
  BrakeSysFeatures : Subsystem
  BrakeSysFeatures_2 : Subsystem
  Bus Creator1 : BusCreator  Inputs=12
  DesiredTorqBrk : Subsystem
  ToCarSim : Subsystem
  WheelData : Subsystem
  WheelSpeed : Subsystem
  Yaw_Data : Subsystem
  Out1 : Outport
  wires:
  Bus Creator1/1 -> Out1/1
  WheelSpeed/1(Out1) -> Bus Creator1/1  "WheelSpeed"
  WheelData/1(Out1) -> Bus Creator1/2  "WheelData"
  BrakeSysFeatures/1(Out1) -> Bus Creator1/8  "BrakeSysFeatures"
  BrakeSnData_4/1(Out1) -> Bus Creator1/7  "BrakeSnData_4"
  DesiredTorqBrk/1(Out1) -> Bus Creator1/6  "DesiredTorqBrk"
  BrakeSnData_3/1(Out1) -> Bus Creator1/5  "BrakeSnData_3"
  Yaw_Data/1(Out1) -> Bus Creator1/4  "Yaw_Data"
  Accel_Data/1(Out1) -> Bus Creator1/3  "Accel_Data"
  In1/1 -> BrakeSysFeatures_2/1(In1), ABS_BrkBst_Data/1(In1), ToCarSim/1(In1), BrakeSnData_5/1(In1), BrakeSysFeatures/1(In1), BrakeSnData_4/1(In1), DesiredTorqBrk/1(In1), BrakeSnData_3/1(In1), Yaw_Data/1(In1), Accel_Data/1(In1), WheelData/1(In1), WheelSpeed/1(In1)
  BrakeSnData_5/1(Out1) -> Bus Creator1/9  "BrakeSnData_5"
  ToCarSim/1(Out1) -> Bus Creator1/10
  ABS_BrkBst_Data/1(Out1) -> Bus Creator1/11  "ABS_BrkBst_Data"
  BrakeSysFeatures_2/1(Out1) -> Bus Creator1/12  "BrakeSysFeatures_2"

== system P702_NI_SoftECU/SoftECU/BCM/Logic ==
  In1 : Inport
  Bus Creator : BusCreator  Inputs=3
  GGCC_Config_Mgmt_ID : Subsystem
  IgnitionState : Subsystem
  OdometerValues : Subsystem
  Out1 : Outport
  wires:
  Bus Creator/1 -> Out1/1  "LogicSignals"
  OdometerValues/1(Out) -> Bus Creator/1
  GGCC_Config_Mgmt_ID/1(Out1) -> Bus Creator/3
  IgnitionState/1(Out) -> Bus Creator/2
  In1/1 -> OdometerValues/1(In), IgnitionState/1(In)

== system P702_NI_SoftECU/SoftECU/BCM/Mapping ==
  In1 : Inport
  BodyEngGateway_2 : Subsystem
  BodyInfo_3 : Subsystem
  Bus Creator : BusCreator  Inputs=7
  Cluster_Info1 : Subsystem
  GGCC_Config_Mgmt_ID : Subsystem
  Gear_Shift_By_Wire : Subsystem
  KeyStates : Subsystem
  Personality_BCM2_Data : Subsystem
  Out1 : Outport
  wires:
  Cluster_Info1/1(Out) -> Bus Creator/2
  BodyInfo_3/1(Out) -> Bus Creator/3
  GGCC_Config_Mgmt_ID/1(Out1) -> Bus Creator/4
  KeyStates/1(Out) -> Bus Creator/1
  In1/1 -> Gear_Shift_By_Wire/1(In1), BodyEngGateway_2/1(In1), GGCC_Config_Mgmt_ID/1(In1), BodyInfo_3/1(In), Cluster_Info1/1(In), KeyStates/1(In)
  Bus Creator/1 -> Out1/1  "MsgSignals"
  BodyEngGateway_2/1(Out1) -> Bus Creator/5
  Gear_Shift_By_Wire/1(Out1) -> Bus Creator/6
  Personality_BCM2_Data/1(Out) -> Bus Creator/7

== system P702_NI_SoftECU/SoftECU/DSMC/Logic ==
  In1 : Inport
  Bus Creator : BusCreator  Inputs=3
  Bus Selector : BusSelector  OutputSignals=DSMC.DrvStatMonData.DrvEngLvlConfid_D_Stat,DSMC.DrvStatMonData.DrvEngageLevel_D_Stat,DSMC.DrvStatMonData.DrvEngageLevel_No_Cnt
  Compute_DrvEngageLevel_No_Cs : Subsystem
  Out1 : Outport
  wires:
  In1/1 -> Bus Selector/1
  Bus Creator/1 -> Out1/1  "LogicSignals"
  Bus Selector/1 -> Bus Creator/1, Compute_DrvEngageLevel_No_Cs/1(DrvEngLvlConfid_D_Stat)  "<DrvEngLvlConfid_D_Stat>"
  Bus Selector/2 -> Compute_DrvEngageLevel_No_Cs/2(DrvEngageLevel_D_Stat)  "<DrvEngageLevel_D_Stat>"
  Bus Selector/3 -> Compute_DrvEngageLevel_No_Cs/3(DrvEngageLevel_No_Cnt)  "<DrvEngageLevel_No_Cnt>"
  Compute_DrvEngageLevel_No_Cs/1(DrvEngageLevel_No_Cs) -> Bus Creator/2  "DrvEngageLevel_No_Cs"
  Compute_DrvEngageLevel_No_Cs/2(DrvEngageLevel_No_Cnt1) -> Bus Creator/3  "DrvEngageLevel_No_Cnt"

== system P702_NI_SoftECU/SoftECU/DSMC/Mapping ==
  In1 : Inport
  Bus Creator : BusCreator  Inputs=1
  DrvStatMonData : Subsystem
  Out1 : Outport
  wires:
  Bus Creator/1 -> Out1/1  "MsgSignals"
  In1/1 -> DrvStatMonData/1(In1)
  DrvStatMonData/1(Out1) -> Bus Creator/1

== system P702_NI_SoftECU/SoftECU/ECM/Logic ==
  In1 : Inport
  Out1 : Outport
  wires:
  In1/1 -> Out1/1

== system P702_NI_SoftECU/SoftECU/ECM/Mapping ==
  In1 : Inport
  CAN : Inport  Port=2
  Bus Creator : BusCreator  Inputs=3
  EngBrakeData : Subsystem
  EngVehicleSpThrottle : Subsystem
  EngVehicleSpThrottle2 : Subsystem
  Out1 : Outport
  wires:
  Bus Creator/1 -> Out1/1  "MsgSignals"
  CAN/1 -> EngBrakeData/1(In1)
  EngVehicleSpThrottle2/1(Out1) -> Bus Creator/1  "EngVehicleSpThrottle2"
  EngBrakeData/1(Out1) -> Bus Creator/2  "EngBrakeData"
  EngVehicleSpThrottle/1(Out1) -> Bus Creator/3  "EngVehicleSpThrottle"
  In1/1 -> EngBrakeData/2(In2), EngVehicleSpThrottle/1(In1), EngVehicleSpThrottle2/1(In2)

== system P702_NI_SoftECU/SoftECU/MRR/Logic ==
  In1 : Inport
  Array2Bus : Subsystem
  Bus2Array : Subsystem
  S-Function Builder : S-Function  InitFcn=try, set_param(gcb,'FunctionName','MapRadarSignals_NI'), end  FunctionName=MapRadarSignals_NI  SFunctionModules=MapRadarSignals_NI_wrapper  SFunctionDeploymentMode=off  EnableBusSupport=off  mask(S-Function Builder){}
      mask help: Simulink:masks:SFunctionBuilder_MD
      mask init:
      | val = [[.9  0.75 0.75 1 1 .9 .9 1]',[1 1 0.75 0.75 .9 .9 1 .9]'];try , sys = get_param(gcb,'SfunBuilderFcnName');if isempty(sys), sys = get_param(gcb,'FunctionName'); end,catch, sys = get_param(gcb,'FunctionName'); end
      settings: CopyFcn=set_param(gcbh,'LinkStatus','none')  PreSaveFcn=try, set_param(gcb,'FunctionName','MapRadarSignals_NI'), end  OpenFcn=sfunctionwizard(gcbh)
      mask Display: plot(val(:,1),val(:,2)),disp(sys), port_label('input',1,'Dist_Fellows'), port_label('input',2,'v_Rel_Fellos'), port_label('input',3,'Angle_Hor_Rel_Fellows'), port_label('output',1,'MappedData'), port_label('output',2,'NumberOfDetections')
  Out1 : Outport
  wires:
  In1/1 -> Bus2Array/1(RadarSensor)
  Bus2Array/1(Dist_Fellows) -> S-Function Builder/1
  Bus2Array/2(v_Rel_Fellows) -> S-Function Builder/2
  Bus2Array/3(Angle_Hor_Rel_Fellows) -> S-Function Builder/3
  S-Function Builder/1 -> Array2Bus/1(MappedData)
  Array2Bus/1(MRR_Data) -> Out1/1
  S-Function Builder/2 -> Array2Bus/2(NumOfDetections)

== system P702_NI_SoftECU/SoftECU/MRR/Mapping ==
  In1 : Inport
  Out1 : Outport
  wires:
  In1/1 -> Out1/1
